simulink model "sampleModel360"  (R2021b)
settings: Solver=VariableStepAuto  StartTime=0.0  StopTime=10.0  RelTol=1e-3
undefined symbols (not defined in the file or in its folder): Newton, Raphson
libraries: simulink x4, slpidlib x1
settings Model: Creator=user  LastModifiedBy=user

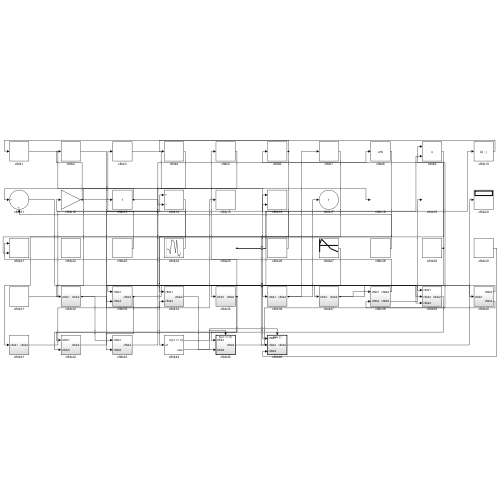
[thumbnail: Simulink's stored preview of the top-level diagram]
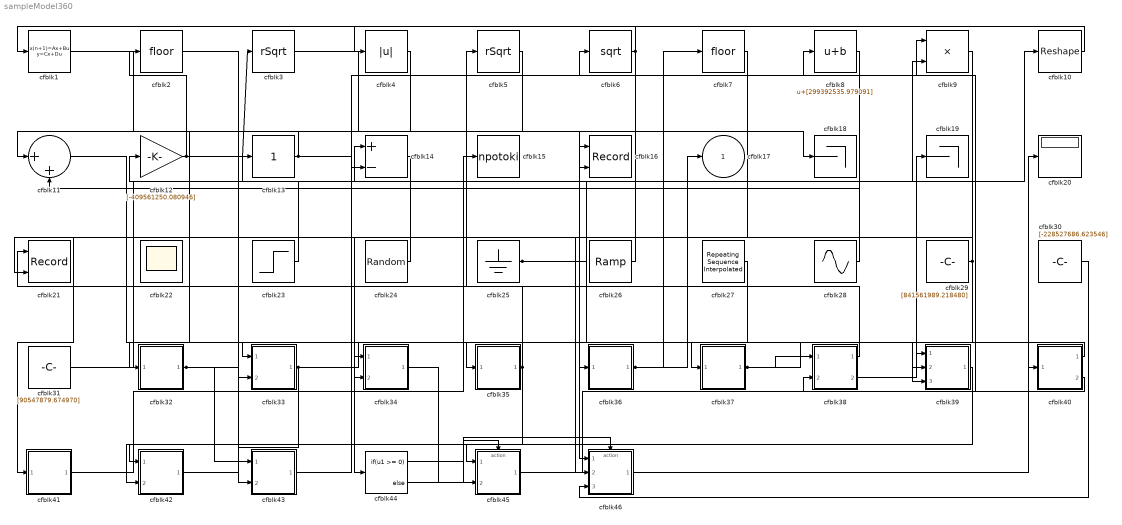
== system sampleModel360 ==
  cfblk1 : DiscreteStateSpace
  cfblk10 : Reshape
  cfblk11 : Sum  Inputs=|++
  cfblk12 : Gain  Gain=[-409561250.080946]
  cfblk13 : simulink/Math Operations/Slider Gain  gain=1  low=0  high=2
  cfblk14 : Sum  Inputs=+-
  cfblk15 : ToWorkspace  VariableName=npotoki  SaveFormat=Timeseries  SampleTime=-1
  cfblk16 : Record  FileSettingsInternal="{\"entries\":[{\"content\":{\"excelSettings\":{\"content\":{},\"type\":\"Streamout.ExcelSettings\"}},\"type\":\"Streamout.FileSettingStorage\",\"uuid\":\"d8db8795-8d82-48a2-b9fa-9258ab88e3d3\"}],\"packageUris\":[\"http://schema.mathworks.com/mf0/streamout_blocks/R2020a\"],\"version\":\"1.0\"}"  Layout=[1 1]  SignalsInternal="{\"entries\":[{\"content\":{\"signals\":[{\"content\":{\"blockPath\":[\"sampleModel360/cfblk16\"],\"channel\":[],\"dimensions\":[1],\"domain\":\"sampleModel360/cfblk16\",\"lineColor\":\"#a2142f\",\"plots\":[1],\"port\":1,\"sid\":[\"\"],\"signalID\":14935,\"signalName\":\"cfblk26\"},\"type\":\"RecordBlkView.Signal\",\"uuid\":\"9002fdfe-f673-40b1-9e75-376e366d3f4b\"},{\"content\":{\"blockPath\":[\"sampleModel360/cfblk16\"],\"channel\":[],\"dimensions\":[1],\"domain\":\"sampleModel360/cfblk16\",\"lineColor\":\"#139fff\",\"plots\":[1],\"port\":2,\"sid\":[\"\"],\"signalID\":14939,\"signalName\":\"cfblk42\"},\"type\":\"RecordBlkView.Signal\",\"uuid\":\"2a6a5ef2-bc7b-4e9e-addd-0580ed7f911f\"}]},\"type\":\"RecordBlkView.InputSignals\",\"uuid\":\"efbb749f-df5f-44e1-8846-bb75c8a8c95a\"}],\"packageUris\":[\"http://schema.mathworks.com/mf0/streamout_blocks/R2020a\"],\"version\":\"1.0\"}"  VisualizationBindings="{\"xyplotplugin\":{\"info\":[{\"series\":[{\"bindingParametersList\":[{\"parameter\":\"X-Axis\",\"signalID\":14935,\"signalName\":\"cfblk26\"},{\"parameter\":\"Y-Axis\",\"signalID\":14939,\"signalName\":\"cfblk42\"}],\"seriesID\":2609}],\"subplotID\":1}]}}"  CompatibilityTag=XY
  cfblk18 : Terminator
  cfblk19 : Terminator
  cfblk2 : Rounding
  cfblk20 : Display
  cfblk21 : Record  FileSettingsInternal="{\"entries\":[{\"content\":{\"excelSettings\":{\"content\":{},\"type\":\"Streamout.ExcelSettings\"}},\"type\":\"Streamout.FileSettingStorage\",\"uuid\":\"a40e61cf-6182-4dd8-ba64-782abd0d7469\"}],\"packageUris\":[\"http://schema.mathworks.com/mf0/streamout_blocks/R2020a\"],\"version\":\"1.0\"}"  Layout=[1 1]  SignalsInternal="{\"entries\":[{\"content\":{\"signals\":[{\"content\":{\"blockPath\":[\"sampleModel360/cfblk21\"],\"channel\":[],\"dimensions\":[1],\"domain\":\"sampleModel360/cfblk21\",\"lineColor\":\"#a2142f\",\"plots\":[1],\"port\":1,\"sid\":[\"\"],\"signalID\":14943,\"signalName\":\"cfblk35\"},\"type\":\"RecordBlkView.Signal\",\"uuid\":\"404e5abb-18d9-4844-9b5f-3b343996f1de\"},{\"content\":{\"blockPath\":[\"sampleModel360/cfblk21\"],\"channel\":[],\"dimensions\":[1],\"domain\":\"sampleModel360/cfblk21\",\"lineColor\":\"#139fff\",\"plots\":[1],\"port\":2,\"sid\":[\"\"],\"signalID\":14947,\"signalName\":\"cfblk9\"},\"type\":\"RecordBlkView.Signal\",\"uuid\":\"8a0c6c16-6498-4bba-abc4-4e1d0acbc8a0\"}]},\"type\":\"RecordBlkView.InputSignals\",\"uuid\":\"d0038ca7-6860-435a-9228-7e06e855bcbb\"}],\"packageUris\":[\"http://schema.mathworks.com/mf0/streamout_blocks/R2020a\"],\"version\":\"1.0\"}"  VisualizationBindings="{\"xyplotplugin\":{\"info\":[{\"series\":[{\"bindingParametersList\":[{\"parameter\":\"X-Axis\",\"signalID\":14943,\"signalName\":\"cfblk35\"},{\"parameter\":\"Y-Axis\",\"signalID\":14947,\"signalName\":\"cfblk9\"}],\"seriesID\":64178}],\"subplotID\":1}]}}"  CompatibilityTag=XY
  cfblk22 : Scope
      settings: Floating=on
  cfblk23 : Step  Time=[11.000000]  Before=[-223864140.613596]  After=[28047343.270318]  SampleTime=0
  cfblk24 : RandomNumber  Mean=[-59313.064769]  Variance=[68202.943447]  Seed=[94317625.000000]  SampleTime=0.1
  cfblk25 : Ground
  cfblk26 : simulink/Sources/Ramp  slope=[4129.850322]  start=[46.616658]  InitialOutput=[892326.872797]
  cfblk27 : simulink/Sources/Repeating Sequence Interpolated  OutValues=[219251237.885766, 868547978.639125, -167755863.699136, -481091997.721669, -905639840.430817]  TimeValues=[0 0.1 0.5 0.6 1].'  LookUpMeth=Interpolation-Use End Values  tsamp=0.01  OutMin=[]  OutMax=[]  OutDataTypeStr=double  OutputDataTypeScalingMode=double  OutDataType=fixdt(0,8)  OutScaling=2^-10
  cfblk28 : Sin  Amplitude=[70892516.327711]  Bias=[778166403.575773]  SampleTime=0
  cfblk29 : Constant  Value=[841561989.218480]  SampleTime=1
  cfblk3 : Sqrt  Operator=rSqrt  AlgorithmType=Newton-Raphson  SaturateOnIntegerOverflow=on
  cfblk30 : Constant  Value=[-228527686.623546]  SampleTime=1
  cfblk31 : Constant  Value=[90547879.674970]  SampleTime=1
  cfblk32 : Subsystem
  cfblk33 : Subsystem
  cfblk34 : Subsystem
  cfblk35 : Subsystem
  cfblk36 : Subsystem
  cfblk37 : Subsystem
  cfblk38 : Subsystem
  cfblk39 : Subsystem
  cfblk4 : Abs
  cfblk40 : Subsystem
  cfblk41 : Subsystem
  cfblk42 : Subsystem
  cfblk43 : Subsystem
  cfblk44 : If  IfExpression=u1 >= 0  SampleTime=1
  cfblk45 : Subsystem  TreatAsAtomicUnit=on
  cfblk46 : Subsystem  TreatAsAtomicUnit=on
  cfblk5 : Sqrt  Operator=rSqrt  AlgorithmType=Newton-Raphson  SaturateOnIntegerOverflow=on
  cfblk6 : Sqrt  SaturateOnIntegerOverflow=on
  cfblk7 : Rounding
  cfblk8 : Bias  Bias=[299392535.979091]
  cfblk9 : Product
  cfblk17 : Outport
  wires:
  cfblk37/1(cfblk2) -> cfblk38/1(cfblk1), cfblk39/1(cfblk1)
  cfblk13/1 -> cfblk11/1, cfblk39/2(cfblk3)
  cfblk7/1 -> cfblk44/1
  cfblk28/1 -> cfblk11/2
  cfblk33/1(cfblk2) -> cfblk37/1(cfblk1), cfblk43/2(cfblk5)
  cfblk29/1 -> cfblk33/1(cfblk1), cfblk6/1
  cfblk43/1(cfblk2) -> cfblk8/1
  cfblk45/1(cfblk2) -> cfblk9/1
  cfblk12/1 -> cfblk3/1, cfblk2/1
  cfblk46/1(cfblk2) -> cfblk20/1
  cfblk35/1(cfblk2) -> cfblk21/1, cfblk42/1(cfblk1), cfblk42/2(cfblk5)
  cfblk9/1 -> cfblk21/2
  cfblk23/1 -> cfblk12/1
  cfblk36/1(cfblk2) -> cfblk17/1, cfblk7/1
  cfblk27/1 -> cfblk33/2(cfblk3)
  cfblk39/1(cfblk2) -> cfblk45/1(cfblk1)
  cfblk38/1(cfblk2) -> cfblk5/1
  cfblk25/1 -> cfblk10/1, cfblk9/2, cfblk39/3(cfblk4)
  cfblk31/1 -> cfblk14/1
  cfblk34/1(cfblk2) -> cfblk45/2(cfblk4)
  cfblk4/1 -> cfblk32/1(cfblk1)
  cfblk14/1 -> cfblk41/1(cfblk1)
  cfblk3/1 -> cfblk46/1(cfblk1)
  cfblk2/1 -> cfblk36/1(cfblk1)
  cfblk10/1 -> cfblk4/1
  cfblk6/1 -> cfblk1/1, cfblk34/1(cfblk1)
  cfblk32/1(cfblk2) -> cfblk43/1(cfblk1), cfblk34/2(cfblk4)
  cfblk40/1(cfblk2) -> cfblk35/1(cfblk1)
  cfblk41/1(cfblk2) -> cfblk15/1
  cfblk1/1 -> cfblk18/1
  cfblk8/1 -> cfblk46/2(cfblk3)
  cfblk40/2(cfblk4) -> cfblk38/2(cfblk4)
  cfblk11/1 -> cfblk40/1(cfblk1)
  cfblk38/2(cfblk5) -> cfblk19/1
  cfblk5/1 -> cfblk14/2
  cfblk26/1 -> cfblk16/1
  cfblk30/1 -> cfblk46/3(cfblk4)
  cfblk42/1(cfblk2) -> cfblk16/2
  cfblk24/1 -> cfblk13/1
  cfblk44/1 -> cfblk45/Action
  cfblk44/2 -> cfblk46/Action

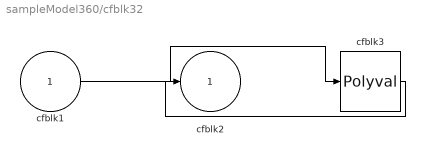
== system sampleModel360/cfblk32 ==
  cfblk1 : Inport
  cfblk3 : Polyval  Coefs=[ +2.081618890e-019, -1.441693666e-014, +4.719686976e-010, -8.536869453e-006, +1.621573104e-001, -8.087801117e+001 ]
  cfblk2 : Outport
  wires:
  cfblk1/1 -> cfblk3/1
  cfblk3/1 -> cfblk2/1

== system sampleModel360/cfblk33 ==
  cfblk1 : Inport
  cfblk3 : Inport  Port=2
  cfblk2 : Outport
  wires:
  cfblk3/1 -> cfblk2/1

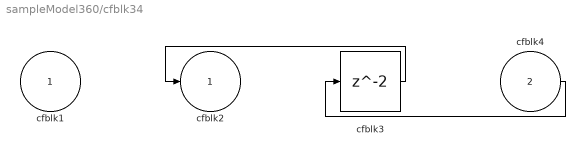
== system sampleModel360/cfblk34 ==
  cfblk1 : Inport
  cfblk4 : Inport  Port=2
  cfblk3 : Delay  SampleTime=1
  cfblk2 : Outport
  wires:
  cfblk3/1 -> cfblk2/1
  cfblk4/1 -> cfblk3/1

== system sampleModel360/cfblk35 ==
  cfblk1 : Inport
  cfblk3 : Constant  Value=[-694521044.975485]  SampleTime=1
  cfblk2 : Outport
  wires:
  cfblk3/1 -> cfblk2/1

== system sampleModel360/cfblk36 ==
  cfblk1 : Inport
  cfblk3 : Product  Inputs=**
  cfblk2 : Outport
  wires:
  cfblk3/1 -> cfblk2/1
  cfblk1/1 -> cfblk3/1, cfblk3/2

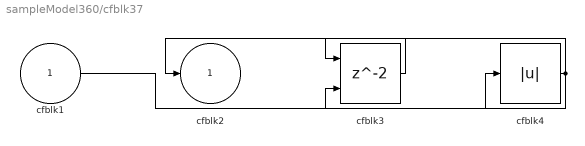
== system sampleModel360/cfblk37 ==
  cfblk1 : Inport
  cfblk3 : Delay  ShowEnablePort=on  SampleTime=1
      settings: InputPortMap=u0,e6
  cfblk4 : Abs
  cfblk2 : Outport
  wires:
  cfblk3/1 -> cfblk2/1
  cfblk1/1 -> cfblk4/1
  cfblk4/1 -> cfblk3/1, cfblk3/2

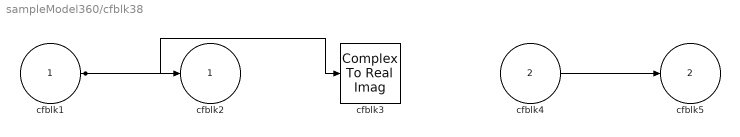
== system sampleModel360/cfblk38 ==
  cfblk1 : Inport
  cfblk4 : Inport  Port=2
  cfblk3 : ComplexToRealImag
  cfblk2 : Outport
  cfblk5 : Outport  Port=2
  wires:
  cfblk1/1 -> cfblk2/1, cfblk3/1
  cfblk4/1 -> cfblk5/1

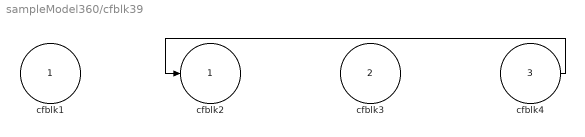
== system sampleModel360/cfblk39 ==
  cfblk1 : Inport
  cfblk3 : Inport  Port=2
  cfblk4 : Inport  Port=3
  cfblk2 : Outport
  wires:
  cfblk4/1 -> cfblk2/1

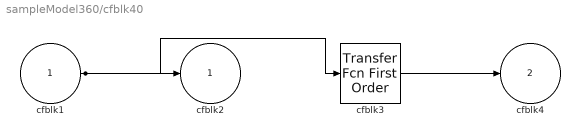
== system sampleModel360/cfblk40 ==
  cfblk1 : Inport
  cfblk3 : simulink/Discrete/Transfer Fcn First Order  PoleZ=0.95  ICPrevOutput=0.0  DoSatur=off
  cfblk2 : Outport
  cfblk4 : Outport  Port=2
  wires:
  cfblk1/1 -> cfblk2/1, cfblk3/1
  cfblk3/1 -> cfblk4/1

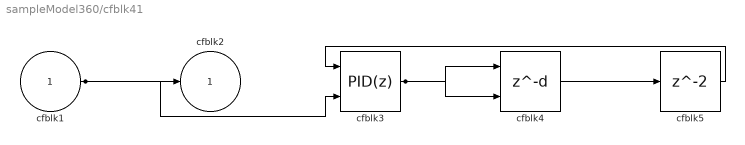
== system sampleModel360/cfblk41 ==
  cfblk1 : Inport
  cfblk3 : slpidlib/PID Controller (2DOF)  Controller=PID  Form=Parallel  TimeDomain=Discrete-time  UseExternalTs=off  SampleTime=1  IntegratorMethod=Forward Euler  FilterMethod=Forward Euler  ControllerParametersSource=internal  P=1  I=1  D=0  UseFilter=on  N=100  b=1  c=1  TunerSelectOption=Transfer Function Based (PID Tuner App)  InitialConditionSource=internal  InitialConditionForIntegrator=0  InitialConditionForFilter=0  DifferentiatorICPrevScaledInput=0  ExternalReset=none  TrackingMode=off  Kt=1  LimitOutput=off  SatLimitsSource=internal  UpperSaturationLimit=inf  LowerSaturationLimit=-inf  LinearizeAsGain=off  AntiWindupMode=none  Kb=1  POutMin=[]  POutMax=[]  IOutMin=[]  IOutMax=[]  DOutMin=[]  DOutMax=[]  NOutMin=[]  NOutMax=[]  bOutMin=[]  bOutMax=[]  cOutMin=[]  cOutMax=[]  SumOutMin=[]  SumOutMax=[]  SaturationOutMin=[]  SaturationOutMax=[]  PParamMin=[]  PParamMax=[]  IParamMin=[]  IParamMax=[]  DParamMin=[]  DParamMax=[]  NParamMin=[]  NParamMax=[]  bParamMin=[]  bParamMax=[]  cParamMin=[]  cParamMax=[]  KbParamMin=[]  KbParamMax=[]  KtParamMin=[]  KtParamMax=[]  KbOutMin=[]  KbOutMax=[]  KtOutMin=[]  KtOutMax=[]  IntegratorOutMin=[]  IntegratorOutMax=[]  FilterOutMin=[]  FilterOutMax=[]  SumI1OutMin=[]  SumI1OutMax=[]  SumI2OutMin=[]  SumI2OutMax=[]  SumI3OutMin=[]  SumI3OutMax=[]  SumI4OutMin=[]  SumI4OutMax=[]  SumDOutMin=[]  SumDOutMax=[]  Sum1OutMin=[]  Sum1OutMax=[]  Sum2OutMin=[]  Sum2OutMax=[]  Sum3OutMin=[]  Sum3OutMax=[]  DifferentiatorOutMin=[]  DifferentiatorOutMax=[]  FilterDiffOutCoefMin=[]  FilterDiffOutCoefMax=[]  ReciprocalOutMin=[]  ReciprocalOutMax=[]  SumDenOutMin=[]  SumDenOutMax=[]  SumNumOutMin=[]  SumNumOutMax=[]  DivideOutMin=[]  DivideOutMax=[]  UdiffTsProdOutMin=[]  UdiffTsProdOutMax=[]  NTsProdOutMin=[]  NTsProdOutMax=[]  UintegralTsProdOutMin=[]  UintegralTsProdOutMax=[]  UngainTsProdOutMin=[]  UngainTsProdOutMax=[]  IntegratorContinuousStateAttributes=''  IntegratorStateMustResolveToSignalObject=off  IntegratorRTWStateStorageClass=Auto  FilterContinuousStateAttributes=''  FilterStateMustResolveToSignalObject=off  FilterRTWStateStorageClass=Auto  ParallelPVariant=InternalParameters  IdealPVariant=Disabled  IVariant=InternalParameters  DVariant=InternalParameters  bVariant=InternalParameters  cVariant=InternalParameters  IntegratorVariant=Discrete  SatVariant=Disabled  AWVariant=Passthrough  PCopyVariant=Disabled  TRVariant=Disabled  FdbkBlocksVariant=Forward  IdealPFdbkVariant=Disabled  SatFdbkVariant=Disabled  DerivativeFilterVariant=ForwardEulerFilter  NVariant=InternalParameters  NCopyVariant=Disabled  FilterICVariant=InternalICsFilter  IntegratorICVariant=InternalICs  ExternalResetVariant=Disabled  TRSumVariant=Passthrough  SumFdbkVariant=Disabled  SumVariant=Sum_PID  TsampFilterVariant=InternalTs  TsampNgainVariant=Passthrough  TsampIntegralVariant=Passthrough  ExternalSaturationOutDataTypeStr=Inherit: Same as second input
      settings: SourceProductBaseCode=SL
  cfblk4 : Delay  DelayLengthSource=Input port  SampleTime=1
      settings: InputPortMap=u0,p1
  cfblk5 : Delay  SampleTime=1
  cfblk2 : Outport
  wires:
  cfblk1/1 -> cfblk2/1, cfblk3/2
  cfblk3/1 -> cfblk4/1, cfblk4/2
  cfblk4/1 -> cfblk5/1
  cfblk5/1 -> cfblk3/1

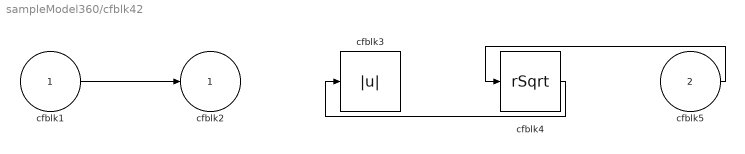
== system sampleModel360/cfblk42 ==
  cfblk1 : Inport
  cfblk5 : Inport  Port=2
  cfblk3 : Abs
  cfblk4 : Sqrt  Operator=rSqrt  AlgorithmType=Newton-Raphson  SaturateOnIntegerOverflow=on
  cfblk2 : Outport
  wires:
  cfblk1/1 -> cfblk2/1
  cfblk5/1 -> cfblk4/1
  cfblk4/1 -> cfblk3/1

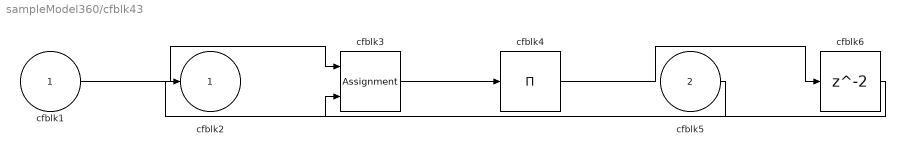
== system sampleModel360/cfblk43 ==
  cfblk1 : Inport
  cfblk5 : Inport  Port=2
  cfblk3 : Assignment  DiagnosticForDimensions=Warning  IndexOptions=Index vector (dialog)  Indices=1  OutputSizes=1
  cfblk4 : Product  Inputs=*
  cfblk6 : Delay  SampleTime=1
  cfblk2 : Outport
  wires:
  cfblk1/1 -> cfblk3/1
  cfblk5/1 -> cfblk2/1
  cfblk3/1 -> cfblk4/1
  cfblk4/1 -> cfblk6/1
  cfblk6/1 -> cfblk3/2

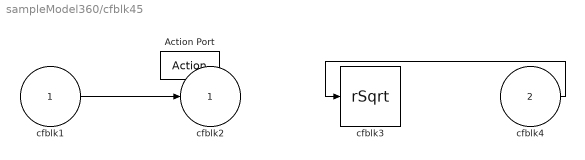
== system sampleModel360/cfblk45 ==
  cfblk1 : Inport
  cfblk4 : Inport  Port=2
  Action Port : ActionPort  ActionPortLabel=if(u1 >= 0)
  cfblk3 : Sqrt  Operator=rSqrt  AlgorithmType=Newton-Raphson  SaturateOnIntegerOverflow=on
  cfblk2 : Outport
  wires:
  cfblk4/1 -> cfblk3/1
  cfblk1/1 -> cfblk2/1

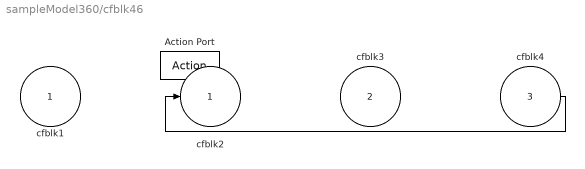
== system sampleModel360/cfblk46 ==
  cfblk1 : Inport
  cfblk3 : Inport  Port=2
  cfblk4 : Inport  Port=3
  Action Port : ActionPort  ActionPortLabel=else
  cfblk2 : Outport
  wires:
  cfblk4/1 -> cfblk2/1
